simulink model "Simulink_Observation_5"  (R2020b)
settings: Solver=VariableStepAuto  StartTime=0.0  StopTime=0  RelTol=1e-3
settings Model: Creator=Mohit Akhouri  LastModifiedBy=Mohit Akhouri

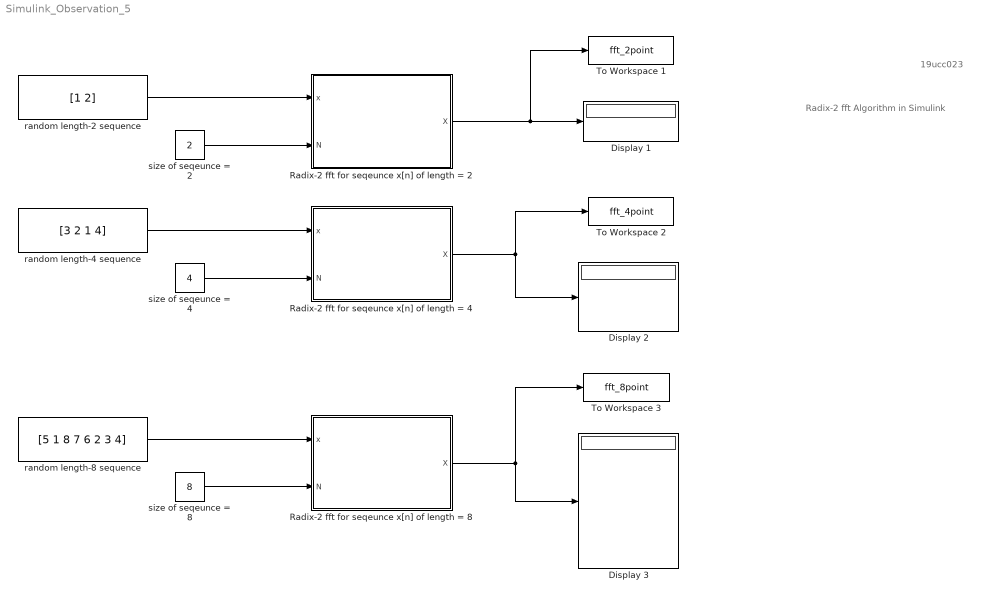
== system Simulink_Observation_5 ==
  note: Radix-2 fft Algorithm in Simulink
  note: 19ucc023
  Display 1 : Display
  Display 2 : Display
  Display 3 : Display
  Radix-2 fft for seqeunce x[n] of length = 2 : MATLAB Function  TreatAsAtomicUnit=on
  Radix-2 fft for seqeunce x[n] of length = 4 : MATLAB Function  TreatAsAtomicUnit=on
  Radix-2 fft for seqeunce x[n] of length = 8 : MATLAB Function  TreatAsAtomicUnit=on
  To Workspace 1 : ToWorkspace  VariableName=fft_2point  SaveFormat=Timeseries  SampleTime=-1
  To Workspace 2 : ToWorkspace  VariableName=fft_4point  SaveFormat=Timeseries  SampleTime=-1
  To Workspace 3 : ToWorkspace  VariableName=fft_8point  SaveFormat=Timeseries  SampleTime=-1
  random length-2 sequence : Constant  Value=[1 2]
  random length-4 sequence : Constant  Value=[3 2 1 4]
  random length-8 sequence : Constant  Value=[5 1 8 7 6 2 3 4]
  size of seqeunce = 2 : Constant  Value=2
  size of seqeunce = 4 : Constant  Value=4
  size of seqeunce = 8 : Constant  Value=8
  wires:
  random length-2 sequence/1 -> Radix-2 fft for seqeunce x[n] of length = 2/1(x)
  size of seqeunce = 2/1 -> Radix-2 fft for seqeunce x[n] of length = 2/2(N)
  Radix-2 fft for seqeunce x[n] of length = 2/1(X) -> To Workspace 1/1, Display 1/1
  random length-4 sequence/1 -> Radix-2 fft for seqeunce x[n] of length = 4/1(x)
  size of seqeunce = 4/1 -> Radix-2 fft for seqeunce x[n] of length = 4/2(N)
  Radix-2 fft for seqeunce x[n] of length = 4/1(X) -> Display 2/1, To Workspace 2/1
  Radix-2 fft for seqeunce x[n] of length = 8/1(X) -> Display 3/1, To Workspace 3/1
  random length-8 sequence/1 -> Radix-2 fft for seqeunce x[n] of length = 8/1(x)
  size of seqeunce = 8/1 -> Radix-2 fft for seqeunce x[n] of length = 8/2(N)

== matlab function Simulink_Observation_5/Radix-2 fft for seqeunce x[n] of length = 2 ==
  data: x input; X output; N input
function X = fcn(x,N)

% 19ucc023
% Mohit Akhouri

X = complex(zeros(1,2));
f1 = complex(zeros(1,N/2)); % To store the ODD parts of sequence x[n]
f2 = complex(zeros(1,N/2)); % To store the EVEN parts of sequence x[n]
Wn = exp(-1j*2*pi/N); % Twiddle factor used in the calculation of DFT

% Main loop algorithm for calculation of DFT via Radix-2 FFT algorithm
for k=1:N/2
    for m=1:N/2
        f1(k) = f1(k) + (x(2*(m-1)+1)*(Wn^(2*(m-1)*(k-1)))); % Calculation of N/2 point-DFT of ODD parts of seqeunce x[n]
        f2(k) = f2(k) + (x(2*(m-1)+2)*(Wn^(2*(m-1)*(k-1)))); % Calculation of N/2 point-DFT of EVEN parts of seqeunce x[n]
    end
    X(k)     = f1(k) + (f2(k)*(Wn^(k-1))); % Combination of f1(k) and f2(k) for N-point DFT of the first half of seqeunce x[n]
    X(k+N/2) = f1(k) - (f2(k)*(Wn^(k-1))); % Combination of f1(k) and f2(k) for N-point DFT of the second half of seqeunce x[n]
end

== matlab function Simulink_Observation_5/Radix-2 fft for seqeunce x[n] of length = 8 ==
  data: x input; X output; N input
function X = fcn(x,N)

% 19ucc023
% Mohit Akhouri

X = complex(zeros(1,8));
f1 = complex(zeros(1,N/2)); % To store the ODD parts of sequence x[n]
f2 = complex(zeros(1,N/2)); % To store the EVEN parts of sequence x[n]
Wn = exp(-1j*2*pi/N); % Twiddle factor used in the calculation of DFT

% Main loop algorithm for calculation of DFT via Radix-2 FFT algorithm
for k=1:N/2
    for m=1:N/2
        f1(k) = f1(k) + (x(2*(m-1)+1)*(Wn^(2*(m-1)*(k-1)))); % Calculation of N/2 point-DFT of ODD parts of seqeunce x[n]
        f2(k) = f2(k) + (x(2*(m-1)+2)*(Wn^(2*(m-1)*(k-1)))); % Calculation of N/2 point-DFT of EVEN parts of seqeunce x[n]
    end
    X(k)     = f1(k) + (f2(k)*(Wn^(k-1))); % Combination of f1(k) and f2(k) for N-point DFT of the first half of seqeunce x[n]
    X(k+N/2) = f1(k) - (f2(k)*(Wn^(k-1))); % Combination of f1(k) and f2(k) for N-point DFT of the second half of seqeunce x[n]
end

== matlab function Simulink_Observation_5/Radix-2 fft for seqeunce x[n] of length = 4 ==
  data: x input; X output; N input
function X = fcn(x,N)

% 19ucc023
% Mohit Akhouri

X = complex(zeros(1,4));
f1 = complex(zeros(1,N/2)); % To store the ODD parts of sequence x[n]
f2 = complex(zeros(1,N/2)); % To store the EVEN parts of sequence x[n]
Wn = exp(-1j*2*pi/N); % Twiddle factor used in the calculation of DFT

% Main loop algorithm for calculation of DFT via Radix-2 FFT algorithm
for k=1:N/2
    for m=1:N/2
        f1(k) = f1(k) + (x(2*(m-1)+1)*(Wn^(2*(m-1)*(k-1)))); % Calculation of N/2 point-DFT of ODD parts of seqeunce x[n]
        f2(k) = f2(k) + (x(2*(m-1)+2)*(Wn^(2*(m-1)*(k-1)))); % Calculation of N/2 point-DFT of EVEN parts of seqeunce x[n]
    end
    X(k)     = f1(k) + (f2(k)*(Wn^(k-1))); % Combination of f1(k) and f2(k) for N-point DFT of the first half of seqeunce x[n]
    X(k+N/2) = f1(k) - (f2(k)*(Wn^(k-1))); % Combination of f1(k) and f2(k) for N-point DFT of the second half of seqeunce x[n]
end
